simulink library "EMACE_APP"  (R2021b)
settings: Solver=VariableStepAuto  StartTime=0.0  StopTime=10.0  RelTol=1e-3
values from neighbouring files (symbols this model uses):
  dataAEMACE = 60.0    [applicationDD.sldd]    (also in dataAEMACE.mat = ; dataAEMACE_DD.sldd)
  sampleTime = 0.008    [applicationDD.sldd]    (also in sampleTime.mat = ; sampleTimeDD.sldd = 0.001
libraries: simulink x2
settings Model: Creator=ACH  LastModifiedBy=ACH

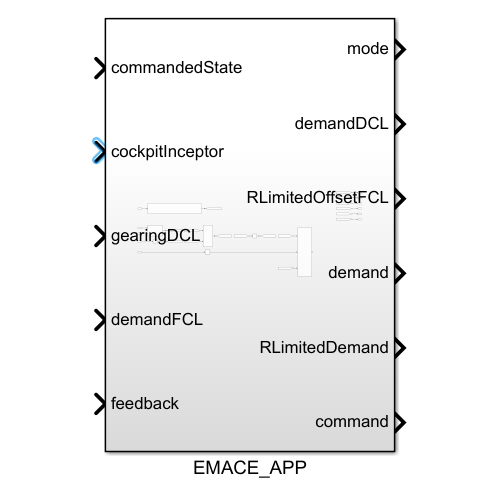
[thumbnail: Simulink's stored preview of the top-level diagram]
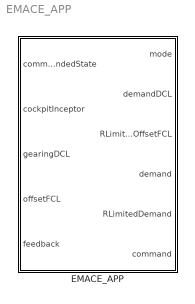
== system EMACE_APP ==
  EMACE_APP : Subsystem

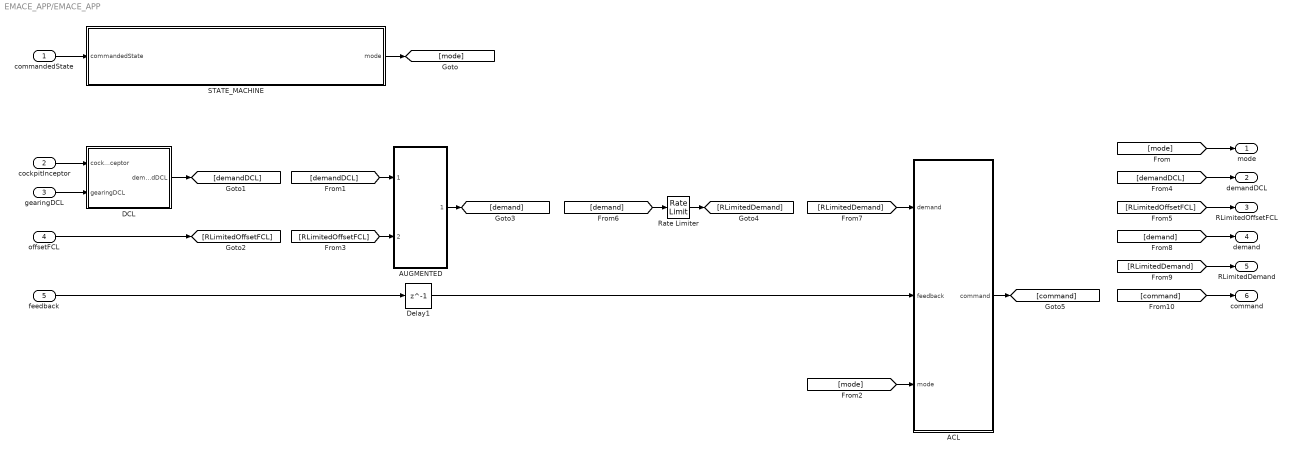
== system EMACE_APP/EMACE_APP ==
  commandedState : Inport
  cockpitInceptor : Inport  Port=2
  gearingDCL : Inport  Port=3
  offsetFCL : Inport  Port=4
  feedback : Inport  Port=5
  ACL : Subsystem
  AUGMENTED : Subsystem
  DCL : Subsystem
  Delay1 : Delay  DelayLength=1  SampleTime=sampleTime.digital
  Rate Limiter : RateLimiter  RisingSlewLimit=dataAEMACE.rateLimiterDemand  FallingSlewLimit=-dataAEMACE.rateLimiterDemand  SampleTimeMode=inherited
      settings: AttributesFormatString=|
      | %<RisingSlewLimit>
      | %<FallingSlewLimit>
  STATE_MACHINE : Subsystem
  mode : Outport
  demandDCL : Outport  Port=2
  RLimitedOffsetFCL : Outport  Port=3
  demand : Outport  Port=4
  RLimitedDemand : Outport  Port=5
  command : Outport  Port=6
  wires:
  [mode] -> ACL/3(mode)
  feedback/1 -> Delay1/1
  gearingDCL/1 -> DCL/2(gearingDCL)
  cockpitInceptor/1 -> DCL/1(cockpitInceptor)
  STATE_MACHINE/1(mode) -> [mode]
  commandedState/1 -> STATE_MACHINE/1(commandedState)
  [mode] -> mode/1
  Delay1/1 -> ACL/2(feedback)
  AUGMENTED/1(demand) -> [demand]
  Rate Limiter/1 -> [RLimitedDemand]
  DCL/1(demandDCL) -> [demandDCL]
  [demandDCL] -> AUGMENTED/1(demandDCL)
  [demandDCL] -> demandDCL/1
  offsetFCL/1 -> [RLimitedOffsetFCL]
  [RLimitedOffsetFCL] -> AUGMENTED/2(demandFCL)
  [RLimitedOffsetFCL] -> RLimitedOffsetFCL/1
  [demand] -> demand/1
  [demand] -> Rate Limiter/1
  [RLimitedDemand] -> ACL/1(demand)
  [RLimitedDemand] -> RLimitedDemand/1
  [command] -> command/1
  ACL/1(command) -> [command]

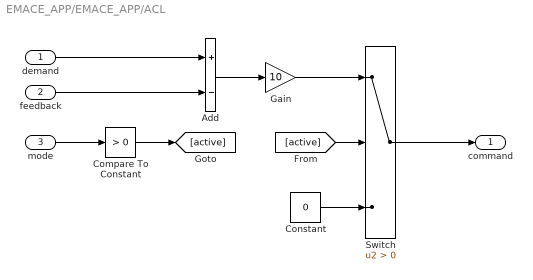
== system EMACE_APP/EMACE_APP/ACL ==
  demand : Inport
  feedback : Inport  Port=2
  mode : Inport  Port=3
  Add : Sum  Inputs=+-
  Compare To Constant : simulink/Logic and Bit Operations/Compare To Constant  relop=>  const=0  OutDataTypeStr=boolean
  Constant : Constant  Value=0
  Gain : Gain  Gain=10
  Switch : Switch  Criteria=u2 > Threshold
  command : Outport  OutDataTypeStr=single
  wires:
  demand/1 -> Add/1
  Add/1 -> Gain/1
  Gain/1 -> Switch/1
  feedback/1 -> Add/2
  mode/1 -> Compare To Constant/1
  Compare To Constant/1 -> [active]
  [active] -> Switch/2
  Constant/1 -> Switch/3
  Switch/1 -> command/1

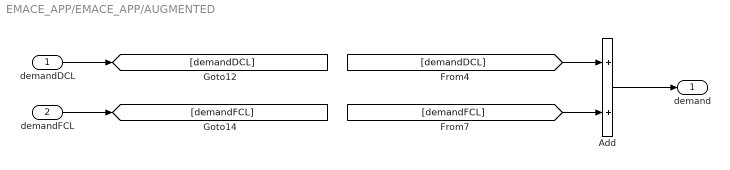
== system EMACE_APP/EMACE_APP/AUGMENTED ==
  demandDCL : Inport
  demandFCL : Inport  Port=2
  Add : Sum
  demand : Outport
  wires:
  [demandDCL] -> Add/1
  [demandFCL] -> Add/2
  demandDCL/1 -> [demandDCL]
  Add/1 -> demand/1
  demandFCL/1 -> [demandFCL]

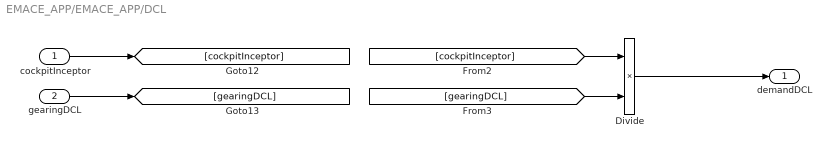
== system EMACE_APP/EMACE_APP/DCL ==
  cockpitInceptor : Inport
  gearingDCL : Inport  Port=2
  Divide : Product  Inputs=**
  demandDCL : Outport
  wires:
  gearingDCL/1 -> [gearingDCL]
  Divide/1 -> demandDCL/1
  [cockpitInceptor] -> Divide/1
  cockpitInceptor/1 -> [cockpitInceptor]
  [gearingDCL] -> Divide/2

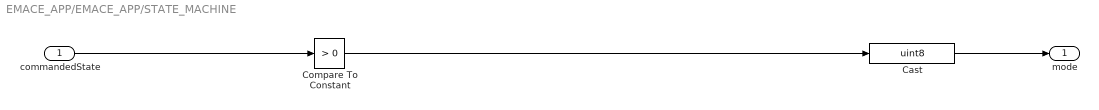
== system EMACE_APP/EMACE_APP/STATE_MACHINE ==
  commandedState : Inport
  Cast : DataTypeConversion  OutDataTypeStr=uint8
  Compare To Constant : simulink/Logic and Bit Operations/Compare To Constant  relop=>  const=0  OutDataTypeStr=boolean
  mode : Outport
  wires:
  Compare To Constant/1 -> Cast/1
  Cast/1 -> mode/1
  commandedState/1 -> Compare To Constant/1
